simulink model "HammingCodeDecoder"  (R2018b)
settings: Solver=FixedStepAuto  StartTime=0.0  StopTime=10.0  RelTol=1e-3
settings Model: Creator=jayakumarav  LastModifiedBy=hiterd

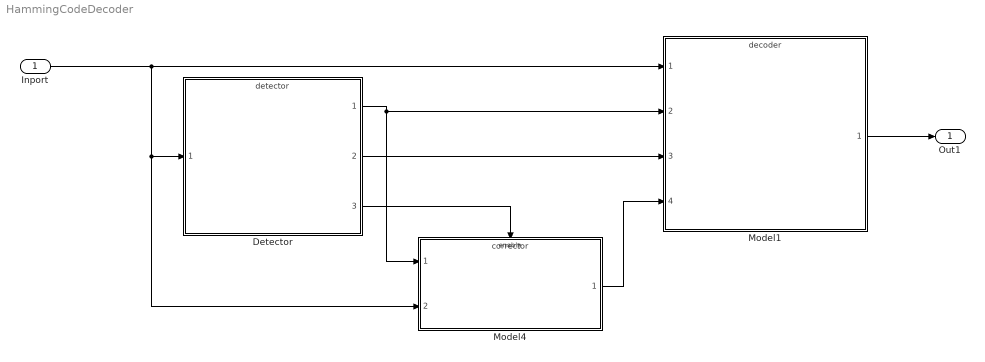
== system HammingCodeDecoder ==
  Inport : Inport
  Detector : ModelReference  ModelNameDialog=detector.slx  SimulationMode=Normal  ModelReferenceVersion=1.29
  Model1 : ModelReference  ModelNameDialog=decoder.slx  SimulationMode=Normal  ModelReferenceVersion=1.32
  Model4 : ModelReference  ModelNameDialog=corrector.slx  SimulationMode=Normal  ModelReferenceVersion=1.7  EnablePortName=Enable  EnablePortStatesWhenEnabling=held
  Out1 : Outport
  wires:
  Detector/1 -> Model4/1, Model1/2
  Detector/3 -> Model4/Enable
  Inport/1 -> Detector/1, Model4/2, Model1/1
  Detector/2 -> Model1/3
  Model4/1 -> Model1/4
  Model1/1 -> Out1/1
